simulink model "FCS_MPC_6ph_testbench_single_test"  (R2022a)
settings: Solver=ode23t  StartTime=0.0  StopTime=0.1  RelTol=1e-3  AbsTol=1e-3  EnableMultiTasking=on
values from neighbouring files (symbols this model uses):
  f_c = 100000    [Params_testbench.m]
  L_d = 0.0001473    [Params_testbench.m]
  L_q = 0.0001484    [Params_testbench.m]
  L_x = 0.00005566    (= 5.566e-05)    [Params_testbench.m]
  L_y = L_x    (= 5.566e-05)    [Params_testbench.m]
  p = 5    [Params_testbench.m]
  psi_pm = 0.0048    [Params_testbench.m]
  R_ph = 0.1278    [Params_testbench.m]
  u_dc = 36.0    (= 36)    [Params_testbench.m]
libraries: nesl_utility x39, fl_lib x32, hdlsllib x26, ee_lib x12, simulink x2, spsAlphaBetaZerotodq0Lib x1
(part 2 of 4)

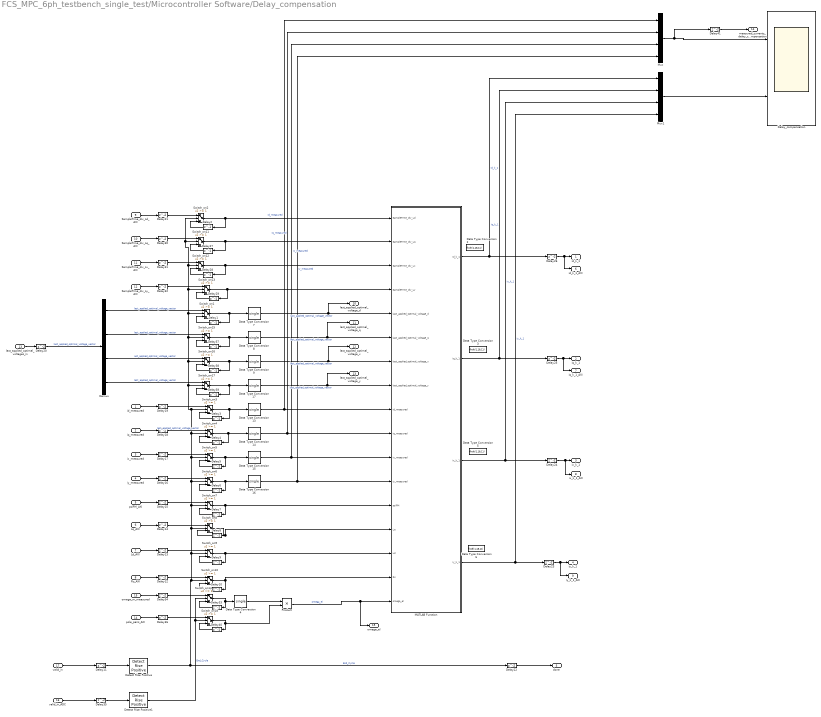
== system FCS_MPC_6ph_testbench_single_test/Microcontroller Software/Delay_compensation ==
  id_measured : Inport
  iq_measured : Inport  Port=2
  ix_measured : Inport  Port=3
  iy_measured : Inport  Port=4
  psiPM_AXI : Inport  Port=5
  Lq_AXI : Inport  Port=6
  Ld_AXI : Inport  Port=7
  Rs_AXI : Inport  Port=8
  SampleTime_div_Ld_AXI : Inport  Port=9
  SampleTime_div_Lq_AXI : Inport  Port=10
  SampleTime_div_Lx_AXI : Inport  Port=11
  SampleTime_div_Ly_AXI : Inport  Port=12
  last_applied_optimal_voltages_in : Inport  Port=13
  pole_pairs_AXI : Inport  Port=14
  omega_m_measured : Inport  Port=15
  valid_in_ADC : Inport  Port=16
  valid_in : Inport  Port=17
  Data Type Conversion{4,7..9,13..17} (9 alike) : DataTypeConversion  OutDataTypeStr=single  RndMeth=Nearest  SaturateOnIntegerOverflow=off
  Data Type Conversion{2..3,5..6} (4 alike) : DataTypeConversion  OutDataTypeStr=fixdt(1,18,11)  SaturateOnIntegerOverflow=off  RndMeth=Floor
  Delay{1..10,27..29,33,37..40} (18 alike) : Delay  DelayLength=1
  Delay{11..26,30..32,34..36,41} (23 alike) : Delay
  Delay_compensation : Scope  NumInputPorts=2
  Demux : Demux
  Detect Rise Positive : hdlsllib/Logic and Bit Operations/Detect Rise Positive  vinit=0  OutDataTypeStr=boolean
      settings: SourceProductBaseCode=SL
  Detect Rise Positive1 : hdlsllib/Logic and Bit Operations/Detect Rise Positive  vinit=0  OutDataTypeStr=boolean
      settings: SourceProductBaseCode=SL
  MATLAB Function : MATLAB Function  TreatAsAtomicUnit=on  SystemSampleTime=1/100000000
  Mux : Mux
  Mux1 : Mux
  Product : Product  Inputs=**
  Switch_on{1..18} (18 alike) : Switch  Threshold=1  RndMeth=Simplest  SaturateOnIntegerOverflow=off  InputSameDT=off  OutDataTypeStr=Inherit: Same as first input
  id_k_1 : Outport
  iq_k_1 : Outport  Port=2
  ix_k_1 : Outport  Port=3
  iy_k_1 : Outport  Port=4
  done : Outport  Port=5
  id_k_1_AXI : Outport  Port=6
  iq_k_1_AXI : Outport  Port=7
  ix_k_1_AXI : Outport  Port=8
  iy_k_1_AXI : Outport  Port=9
  last_applied_optimal_voltage_d : Outport  Port=10
  last_applied_optimal_voltage_q : Outport  Port=11
  last_applied_optimal_voltage_x : Outport  Port=12
  last_applied_optimal_voltage_y : Outport  Port=13
  measured_currents_delay_compensation : Outport  Port=14
  omega_el : Outport  Port=15
  wires:
  Switch_on14/1 -> Data Type Conversion4/1, Delay33/1
  Delay33/1 -> Switch_on14/3
  pole_pairs_AXI/1 -> Delay36/1
  Delay9/1 -> Switch_on9/3
  Switch_on9/1 -> Delay9/1, MATLAB Function/15(Ld)
  Delay32/1 -> Switch_on13/1
  Lq_AXI/1 -> Delay14/1
  Delay31/1 -> Switch_on12/1
  Switch_on12/1 -> Delay28/1, MATLAB Function/3(SampleTime_div_Lx)
  Delay30/1 -> Switch_on11/1
  Delay29/1 -> Switch_on13/3
  SampleTime_div_Lx_AXI/1 -> Delay31/1
  Delay26/1 -> id_k_1_AXI/1, id_k_1/1
  Product/1 -> omega_el/1, MATLAB Function/17(omega_el)  "omega_el"
  Delay11/1 -> Detect Rise Positive/1
  Delay2/1 -> Switch_on2/3
  SampleTime_div_Lq_AXI/1 -> Delay30/1
  Switch_on5/1 -> Delay5/1, Data Type Conversion15/1
  Delay12/1 -> Switch_on10/1
  Rs_AXI/1 -> Delay12/1
  Delay1/1 -> Switch_on1/3
  Delay27/1 -> Switch_on11/3
  Delay21/1 -> Switch_on2/1
  Delay23/1 -> iy_k_1_AXI/1, iy_k_1/1
  Delay24/1 -> ix_k_1_AXI/1, ix_k_1/1
  Delay20/1 -> Demux/1  "last_applied_optimal_voltage_vector"
  Switch_on1/1 -> Delay1/1, Data Type Conversion7/1
  Delay8/1 -> Switch_on8/3
  Delay10/1 -> Switch_on10/3
  valid_in/1 -> Delay11/1
  Switch_on6/1 -> Delay6/1, Data Type Conversion16/1
  psiPM_AXI/1 -> Delay15/1
  Delay25/1 -> iq_k_1_AXI/1, iq_k_1/1
  Switch_on13/1 -> Delay29/1, MATLAB Function/4(SampleTime_div_Ly)
  Switch_on4/1 -> Delay4/1, Data Type Conversion14/1
  Delay15/1 -> Switch_on7/1
  SampleTime_div_Ly_AXI/1 -> Delay32/1
  Switch_on10/1 -> Delay10/1, MATLAB Function/16(Rs)
  Delay7/1 -> Switch_on7/3
  Delay28/1 -> Switch_on12/3
  Switch_on8/1 -> Delay8/1, MATLAB Function/14(Lq)
  Ld_AXI/1 -> Delay13/1
  Delay6/1 -> Switch_on6/3
  Delay4/1 -> Switch_on4/3
  Switch_on11/1 -> Delay27/1, MATLAB Function/2(SampleTime_div_Lq)
  Delay3/1 -> Switch_on3/3
  Delay14/1 -> Switch_on8/1
  Switch_on2/1 -> Delay2/1, MATLAB Function/1(SampleTime_div_Ld)
  Delay22/1 -> done/1
  Switch_on3/1 -> Delay3/1, Data Type Conversion13/1
  Delay13/1 -> Switch_on9/1
  Delay5/1 -> Switch_on5/3
  SampleTime_div_Ld_AXI/1 -> Delay21/1
  last_applied_optimal_voltages_in/1 -> Delay20/1
  id_measured/1 -> Delay19/1
  iq_measured/1 -> Delay18/1
  ix_measured/1 -> Delay17/1
  iy_measured/1 -> Delay16/1
  omega_m_measured/1 -> Delay34/1
  Delay35/1 -> Detect Rise Positive1/1
  valid_in_ADC/1 -> Delay35/1
  Delay34/1 -> Switch_on14/1
  Delay36/1 -> Switch_on18/1
  Delay37/1 -> Switch_on15/3
  Delay38/1 -> Switch_on16/3
  Switch_on16/1 -> Data Type Conversion9/1, Delay38/1
  Delay39/1 -> Switch_on17/3
  Detect Rise Positive/1 -> Switch_on17/2, Switch_on16/2, Switch_on15/2, Switch_on13/2, Switch_on2/2, Switch_on11/2, Switch_on12/2, Switch_on1/2, Switch_on3/2, Switch_on4/2, Switch_on5/2, Switch_on6/2, Switch_on7/2, Switch_on8/2, Switch_on9/2, Switch_on10/2, Delay22/1  "End_Cycle"
  Switch_on17/1 -> Data Type Conversion17/1, Delay39/1
  Delay19/1 -> Switch_on3/1
  Delay18/1 -> Switch_on4/1  "last_applied_optimal_voltage_vector"
  Delay17/1 -> Switch_on5/1
  Delay16/1 -> Switch_on6/1
  Data Type Conversion4/1 -> Product/1
  MATLAB Function/1(id_k_1) -> Mux1/1, Delay26/1  "id_k_1"
  MATLAB Function/2(iq_k_1) -> Mux1/2, Delay25/1  "iq_k_1"
  MATLAB Function/3(ix_k_1) -> Mux1/3, Delay24/1  "ix_k_1"
  MATLAB Function/4(iy_k_1) -> Mux1/4, Delay23/1  "iy_k_1"
  Switch_on18/1 -> Product/2, Delay40/1
  Detect Rise Positive1/1 -> Switch_on18/2, Switch_on14/2  "End_Cycle"
  Delay40/1 -> Switch_on18/3
  Data Type Conversion13/1 -> Mux/1, MATLAB Function/9(id_measured)  "id_measured"
  Data Type Conversion14/1 -> Mux/2, MATLAB Function/10(iq_measured)  "iq_measured"
  Data Type Conversion15/1 -> Mux/3, MATLAB Function/11(ix_measured)  "ix_measured"
  Data Type Conversion16/1 -> Mux/4, MATLAB Function/12(iy_measured)  "iy_measured"
  Switch_on7/1 -> MATLAB Function/13(psiPM), Delay7/1
  Mux/1 -> Delay41/1, Delay_compensation/1
  Mux1/1 -> Delay_compensation/2
  Switch_on15/1 -> Data Type Conversion8/1, Delay37/1
  Demux/1 -> Switch_on1/1  "last_applied_optimal_voltage_vector"
  Demux/2 -> Switch_on15/1  "last_applied_optimal_voltage_vector"
  Demux/3 -> Switch_on16/1  "ast_applied_optimal_voltage_vector"
  Demux/4 -> Switch_on17/1  "last_applied_optimal_voltage_vector"
  Data Type Conversion7/1 -> last_applied_optimal_voltage_d/1, MATLAB Function/5(last_applied_optimal_voltage_d)  "last_applied_optimal_voltage_vector"
  Data Type Conversion8/1 -> last_applied_optimal_voltage_q/1, MATLAB Function/6(last_applied_optimal_voltage_q)  "last_applied_optimal_voltage_vector"
  Data Type Conversion9/1 -> last_applied_optimal_voltage_x/1, MATLAB Function/7(last_applied_optimal_voltage_x)  "last_applied_optimal_voltage_vector"
  Data Type Conversion17/1 -> last_applied_optimal_voltage_y/1, MATLAB Function/8(last_applied_optimal_voltage_y)  "last_applied_optimal_voltage_vector"
  Delay41/1 -> measured_currents_delay_compensation/1

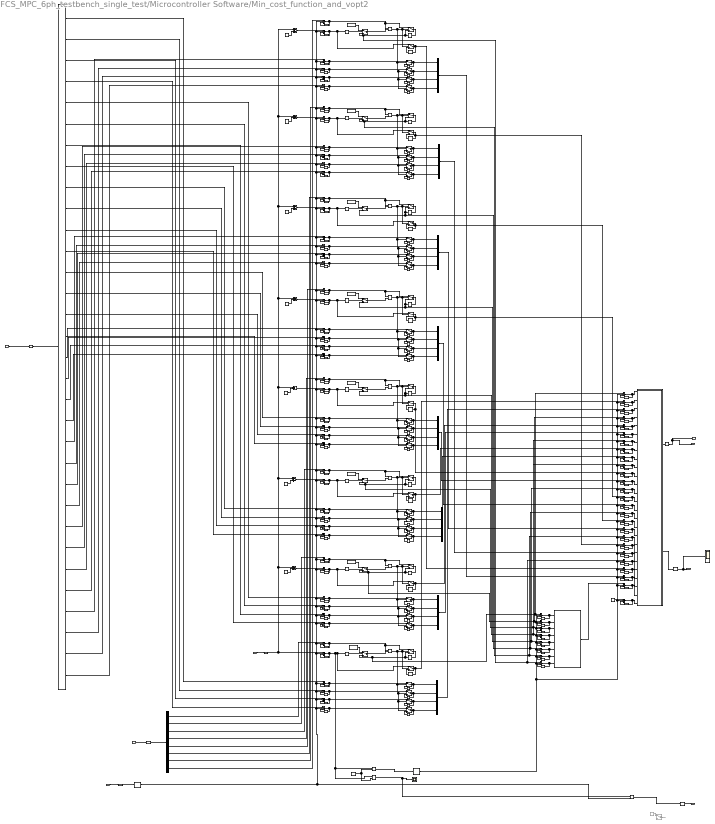
== system FCS_MPC_6ph_testbench_single_test/Microcontroller Software/Min_cost_function_and_vopt2 ==
  note: fixdt(1,24,11)
  Index_in : Inport
  valid_in : Inport  Port=2
  J_in : Inport  Port=3
  phase_voltages_per_switching_state_in : Inport  Port=4
  Add{,1..6} (7 alike) : Sum
  Compare To Constant : hdlsllib/Logic and Bit Operations/Compare To Constant  relop=<=  const=1  OutDataTypeStr=boolean
      settings: SourceProductBaseCode=SL
  Compare To Constant1 : hdlsllib/Logic and Bit Operations/Compare To Constant  relop=<=  const=9  OutDataTypeStr=boolean
      settings: SourceProductBaseCode=SL
  Compare To Constant2 : hdlsllib/Logic and Bit Operations/Compare To Constant  relop=<=  const=17  OutDataTypeStr=boolean
      settings: SourceProductBaseCode=SL
  Compare To Constant3 : hdlsllib/Logic and Bit Operations/Compare To Constant  relop=<=  const=25  OutDataTypeStr=boolean
      settings: SourceProductBaseCode=SL
  Compare To Constant4 : hdlsllib/Logic and Bit Operations/Compare To Constant  relop=<=  const=33  OutDataTypeStr=boolean
      settings: SourceProductBaseCode=SL
  Compare To Constant5 : hdlsllib/Logic and Bit Operations/Compare To Constant  relop=<=  const=41  OutDataTypeStr=boolean
      settings: SourceProductBaseCode=SL
  Compare To Constant6 : hdlsllib/Logic and Bit Operations/Compare To Constant  relop=<=  const=49  OutDataTypeStr=boolean
      settings: SourceProductBaseCode=SL
  Compare To Constant7 : hdlsllib/Logic and Bit Operations/Compare To Constant  relop=<=  const=57  OutDataTypeStr=boolean
      settings: SourceProductBaseCode=SL
  Constant{,3..9} (8 alike) : Constant  Value=1000  OutDataTypeStr=fixdt(1,20,9)  SampleTime=-1
  Constant1 : Constant  Value=8  OutDataTypeStr=int32  SampleTime=-1
  Constant11 : Constant  Value=[0;0;0;0]  OutDataTypeStr=single  SampleTime=-1
  Constant18 : Constant  Value=8  OutDataTypeStr=int32  SampleTime=-1
  Constant19 : Constant  Value=16  OutDataTypeStr=int32  SampleTime=-1
  Constant2 : Constant  Commented=on  Value=0  OutDataTypeStr=boolean  SampleTime=-1
  Constant20 : Constant  Value=24  OutDataTypeStr=int32  SampleTime=-1
  Constant21 : Constant  Value=32  OutDataTypeStr=int32  SampleTime=-1
  Constant22 : Constant  Value=40  OutDataTypeStr=int32  SampleTime=-1
  Constant23 : Constant  Value=48  OutDataTypeStr=int32  SampleTime=-1
  Constant24 : Constant  Value=56  OutDataTypeStr=int32  SampleTime=-1
  Delay{,1..5,9,15,17..73,81..90,95..96,104..113,118..119,127..136,141..142,150..159,164..165,173..182,371..378} (131 alike) : Delay  DelayLength=1
  Delay{6..8,10..12} (6 alike) : Delay
  Delay_compensation_test1 : Scope
  Demux : Demux  Outputs=8
  Demux1 : Demux  Outputs=32
  Detect Rise Positive : hdlsllib/Logic and Bit Operations/Detect Rise Positive  vinit=0  OutDataTypeStr=boolean
      settings: SourceProductBaseCode=SL
  Detect Rise Positive1 : hdlsllib/Logic and Bit Operations/Detect Rise Positive  vinit=0  OutDataTypeStr=boolean
      settings: SourceProductBaseCode=SL
  Logical Operator : Logic  AllPortsSameDT=off  OutDataTypeStr=boolean
  MATLAB Function : MATLAB Function  TreatAsAtomicUnit=on  SystemSampleTime=1/100000000
  MinMax : MinMax  Inputs=8  ZeroCross=off
  Mux{,1..7} (8 alike) : Mux
  Relational Operator{,1..8} (9 alike) : RelationalOperator  Operator=<  OutDataTypeStr=boolean  RndMeth=Simplest  InputSameDT=off
  Relational Operator9 : RelationalOperator  OutDataTypeStr=boolean  RndMeth=Simplest  InputSameDT=off
  Scope : Scope
  Switch{,1,3..6,8..9,11..14,16..21,23..28,30..35,37..42,44..49,51..56} (48 alike) : Switch  Criteria=u2 > Threshold  SaturateOnIntegerOverflow=off  InputSameDT=off  OutDataTypeStr=Inherit: Same as first input
  Switch{2,10,15,22,29,36,43,50} (8 alike) : Switch  Criteria=u2 > Threshold  OutDataTypeStr=int32  SaturateOnIntegerOverflow=off  InputSameDT=off
  Switch7 : Switch  Commented=on  Criteria=u2 > Threshold  SaturateOnIntegerOverflow=off  InputSameDT=off
  Switch_on{1..49,51..75,98..105} (82 alike) : Switch  Threshold=1  RndMeth=Simplest  SaturateOnIntegerOverflow=off  InputSameDT=off  OutDataTypeStr=Inherit: Same as first input
      Switch_on49 settings: LockScale=on
  done : Outport
  Index : Outport  Port=2
  voltages : Outport  Port=3
  Index_AXI : Outport  Port=4
  wires:
  Demux/1 -> Switch_on4/1  "End_Cycle"
  Demux1/1 -> Switch_on2/1  "End_Cycle"
  Demux1/2 -> Switch_on3/1  "End_Cycle"
  Switch5/1 -> Mux/3, Delay4/1
  Delay3/1 -> Switch4/3
  Relational Operator/1 -> Switch5/2, Switch6/2, Switch4/2, Switch3/2, Switch2/2, Switch1/2
  Compare To Constant/1 -> Switch/2
  Switch1/1 -> Delay/1
  Switch6/1 -> Delay5/1, Mux/4
  Delay4/1 -> Switch5/3
  Switch4/1 -> Mux/2, Delay3/1
  Switch/1 -> Relational Operator/2
  Delay1/1 -> Switch2/3
  Delay5/1 -> Switch6/3
  Switch3/1 -> Mux/1, Delay2/1
  Delay2/1 -> Switch3/3
  Constant/1 -> Switch/1
  Switch_on4/1 -> Relational Operator/1, Switch1/1, Delay17/1
  Switch_on1/1 -> Delay18/1, Compare To Constant/1, Switch2/1, Relational Operator9/1, Relational Operator1/1
  Switch_on2/1 -> Delay19/1, Switch3/1
  Switch_on3/1 -> Delay20/1, Switch4/1
  Switch_on5/1 -> Switch5/1, Delay21/1
  Switch_on6/1 -> Switch6/1, Delay22/1
  valid_in/1 -> Delay6/1  "End_Cycle"
  Delay17/1 -> Switch_on4/3
  Delay18/1 -> Switch_on1/3
  Delay19/1 -> Switch_on2/3
  Delay20/1 -> Switch_on3/3
  Delay21/1 -> Switch_on5/3
  Delay22/1 -> Switch_on6/3
  Constant1/1 -> Relational Operator9/2, Relational Operator1/2
  Constant2/1 -> Switch7/1
  Demux1/3 -> Switch_on5/1  "End_Cycle"
  Demux1/4 -> Switch_on6/1  "End_Cycle"
  Demux/2 -> Switch_on10/1  "End_Cycle"
  Delay34/1 -> Switch_on10/3
  Switch8/1 -> Relational Operator2/2
  Switch_on8/1 -> Delay36/1, Switch11/1
  Demux1/6 -> Switch_on9/1  "End_Cycle"
  Delay26/1 -> Switch10/3
  Add/1 -> Switch_on7/1
  Delay36/1 -> Switch_on8/3
  Delay39/1 -> Switch_on11/3
  Switch_on7/1 -> Delay35/1, Switch10/1, Compare To Constant1/1
  Compare To Constant1/1 -> Switch8/2
  Switch_on9/1 -> Delay38/1, Switch12/1
  Delay40/1 -> Switch_on12/3
  Delay35/1 -> Switch_on7/3
  Switch_on11/1 -> Switch13/1, Delay39/1
  Delay43/1 -> Switch14/3
  Switch_on12/1 -> Switch14/1, Delay40/1
  Delay37/1 -> Switch11/3
  Relational Operator2/1 -> Switch13/2, Switch14/2, Switch12/2, Switch11/2, Switch10/2, Switch9/2
  Switch9/1 -> Delay25/1
  Delay42/1 -> Switch13/3
  Demux1/5 -> Switch_on8/1  "End_Cycle"
  Demux1/7 -> Switch_on11/1  "End_Cycle"
  Switch_on10/1 -> Relational Operator2/1, Switch9/1, Delay34/1
  Demux1/8 -> Switch_on12/1  "End_Cycle"
  Delay38/1 -> Switch_on9/3
  Constant3/1 -> Switch8/1
  Delay41/1 -> Switch12/3
  Delay61/1 -> Switch16/3
  Switch_on16/1 -> Switch19/1, Delay64/1
  Delay67/1 -> Switch19/3
  Switch_on15/1 -> Switch18/1, Delay63/1
  Delay59/1 -> Switch_on17/3
  Switch_on19/1 -> Delay62/1, Switch17/1
  Delay64/1 -> Switch_on16/3
  Switch_on17/1 -> Delay59/1, Switch15/1, Compare To Constant2/1
  Compare To Constant2/1 -> Switch20/2
  Demux1/10 -> Switch_on19/1  "End_Cycle"
  Delay50/1 -> Switch15/3
  Switch20/1 -> Relational Operator3/2
  Demux/3 -> Switch_on14/1  "End_Cycle"
  Delay65/1 -> Switch17/3
  Switch_on14/1 -> Relational Operator3/1, Switch21/1, Delay58/1
  Switch_on18/1 -> Delay60/1, Switch16/1
  Constant4/1 -> Switch20/1
  Demux1/11 -> Switch_on15/1  "End_Cycle"
  Delay63/1 -> Switch_on15/3
  Delay66/1 -> Switch18/3
  Switch21/1 -> Delay49/1
  Demux1/9 -> Switch_on18/1  "End_Cycle"
  Demux1/12 -> Switch_on16/1  "End_Cycle"
  Add1/1 -> Switch_on17/1
  Delay60/1 -> Switch_on18/3
  Relational Operator3/1 -> Switch18/2, Switch19/2, Switch17/2, Switch16/2, Switch15/2, Switch21/2
  Delay58/1 -> Switch_on14/3
  Delay62/1 -> Switch_on19/3
  Delay84/1 -> Switch23/3
  Switch_on22/1 -> Switch26/1, Delay87/1
  Delay90/1 -> Switch26/3
  Switch_on21/1 -> Switch25/1, Delay86/1
  Delay82/1 -> Switch_on23/3
  Switch_on25/1 -> Delay85/1, Switch24/1
  Delay87/1 -> Switch_on22/3
  Switch_on23/1 -> Delay82/1, Switch22/1, Compare To Constant3/1
  Compare To Constant3/1 -> Switch27/2
  Demux1/14 -> Switch_on25/1  "End_Cycle"
  Delay73/1 -> Switch22/3
  Switch27/1 -> Relational Operator4/2
  Demux/4 -> Switch_on20/1  "End_Cycle"
  Delay88/1 -> Switch24/3
  Switch_on20/1 -> Relational Operator4/1, Switch28/1, Delay81/1
  Switch_on24/1 -> Delay83/1, Switch23/1
  Constant5/1 -> Switch27/1
  Demux1/15 -> Switch_on21/1  "End_Cycle"
  Delay86/1 -> Switch_on21/3
  Delay89/1 -> Switch25/3
  Switch28/1 -> Delay72/1
  Demux1/13 -> Switch_on24/1  "End_Cycle"
  Demux1/16 -> Switch_on22/1  "End_Cycle"
  Add2/1 -> Switch_on23/1
  Delay83/1 -> Switch_on24/3
  Relational Operator4/1 -> Switch25/2, Switch26/2, Switch24/2, Switch23/2, Switch22/2, Switch28/2
  Delay81/1 -> Switch_on20/3
  Delay85/1 -> Switch_on25/3
  Delay107/1 -> Switch30/3
  Switch_on28/1 -> Switch33/1, Delay110/1
  Delay113/1 -> Switch33/3
  Switch_on27/1 -> Switch32/1, Delay109/1
  Delay105/1 -> Switch_on29/3
  Switch_on31/1 -> Delay108/1, Switch31/1
  Delay110/1 -> Switch_on28/3
  Switch_on29/1 -> Delay105/1, Switch29/1, Compare To Constant4/1
  Compare To Constant4/1 -> Switch34/2
  Demux1/18 -> Switch_on31/1  "End_Cycle"
  Delay96/1 -> Switch29/3
  Switch34/1 -> Relational Operator5/2
  Demux/5 -> Switch_on26/1  "End_Cycle"
  Delay111/1 -> Switch31/3
  Switch_on26/1 -> Relational Operator5/1, Switch35/1, Delay104/1
  Switch_on30/1 -> Delay106/1, Switch30/1
  Constant6/1 -> Switch34/1
  Demux1/19 -> Switch_on27/1  "End_Cycle"
  Delay109/1 -> Switch_on27/3
  Delay112/1 -> Switch32/3
  Switch35/1 -> Delay95/1
  Demux1/17 -> Switch_on30/1  "End_Cycle"
  Demux1/20 -> Switch_on28/1  "End_Cycle"
  Add3/1 -> Switch_on29/1
  Delay106/1 -> Switch_on30/3
  Relational Operator5/1 -> Switch32/2, Switch33/2, Switch31/2, Switch30/2, Switch29/2, Switch35/2
  Delay104/1 -> Switch_on26/3
  Delay108/1 -> Switch_on31/3
  Delay130/1 -> Switch37/3
  Switch_on34/1 -> Switch40/1, Delay133/1
  Delay136/1 -> Switch40/3
  Switch_on33/1 -> Switch39/1, Delay132/1
  Delay128/1 -> Switch_on35/3
  Switch_on37/1 -> Delay131/1, Switch38/1
  Delay133/1 -> Switch_on34/3
  Switch_on35/1 -> Delay128/1, Switch36/1, Compare To Constant5/1
  Compare To Constant5/1 -> Switch41/2
  Demux1/22 -> Switch_on37/1  "End_Cycle"
  Delay119/1 -> Switch36/3
  Switch41/1 -> Relational Operator6/2
  Demux/6 -> Switch_on32/1  "End_Cycle"
  Delay134/1 -> Switch38/3
  Switch_on32/1 -> Relational Operator6/1, Switch42/1, Delay127/1
  Switch_on36/1 -> Delay129/1, Switch37/1
  Constant7/1 -> Switch41/1
  Demux1/23 -> Switch_on33/1  "End_Cycle"
  Delay132/1 -> Switch_on33/3
  Delay135/1 -> Switch39/3
  Switch42/1 -> Delay118/1
  Demux1/21 -> Switch_on36/1  "End_Cycle"
  Demux1/24 -> Switch_on34/1  "End_Cycle"
  Add4/1 -> Switch_on35/1
  Delay129/1 -> Switch_on36/3
  Relational Operator6/1 -> Switch39/2, Switch40/2, Switch38/2, Switch37/2, Switch36/2, Switch42/2
  Delay127/1 -> Switch_on32/3
  Delay131/1 -> Switch_on37/3
  Delay153/1 -> Switch44/3
  Switch_on40/1 -> Switch47/1, Delay156/1
  Delay159/1 -> Switch47/3
  Switch_on39/1 -> Switch46/1, Delay155/1
  Delay151/1 -> Switch_on41/3
  Switch_on43/1 -> Delay154/1, Switch45/1
  Delay156/1 -> Switch_on40/3
  Switch_on41/1 -> Delay151/1, Switch43/1, Compare To Constant6/1
  Compare To Constant6/1 -> Switch48/2
  Demux1/26 -> Switch_on43/1  "End_Cycle"
  Delay142/1 -> Switch43/3
  Switch48/1 -> Relational Operator7/2
  Delay157/1 -> Switch45/3
  Switch_on38/1 -> Relational Operator7/1, Switch49/1, Delay150/1
  Switch_on42/1 -> Delay152/1, Switch44/1
  Constant8/1 -> Switch48/1
  Demux1/27 -> Switch_on39/1  "End_Cycle"
  Delay155/1 -> Switch_on39/3
  Delay158/1 -> Switch46/3
  Switch49/1 -> Delay141/1
  Demux1/25 -> Switch_on42/1  "End_Cycle"
  Demux1/28 -> Switch_on40/1  "End_Cycle"
  Add5/1 -> Switch_on41/1
  Delay152/1 -> Switch_on42/3
  Relational Operator7/1 -> Switch46/2, Switch47/2, Switch45/2, Switch44/2, Switch43/2, Switch49/2
  Delay150/1 -> Switch_on38/3
  Delay154/1 -> Switch_on43/3
  Delay176/1 -> Switch51/3
  Switch_on46/1 -> Switch54/1, Delay179/1
  Delay182/1 -> Switch54/3
  Switch_on45/1 -> Switch53/1, Delay178/1
  Delay174/1 -> Switch_on47/3
  Switch_on49/1 -> Delay177/1, Switch52/1
  Delay179/1 -> Switch_on46/3
  Switch_on47/1 -> Delay174/1, Switch50/1, Compare To Constant7/1
  Compare To Constant7/1 -> Switch55/2
  Demux1/30 -> Switch_on49/1  "End_Cycle"
  Delay165/1 -> Switch50/3
  Switch55/1 -> Relational Operator8/2
  Demux/8 -> Switch_on44/1  "End_Cycle"
  Delay180/1 -> Switch52/3
  Switch_on44/1 -> Relational Operator8/1, Switch56/1, Delay173/1
  Switch_on48/1 -> Delay175/1, Switch51/1
  Constant9/1 -> Switch55/1
  Demux1/31 -> Switch_on45/1  "End_Cycle"
  Delay178/1 -> Switch_on45/3
  Delay181/1 -> Switch53/3
  Switch56/1 -> Delay164/1
  Demux1/29 -> Switch_on48/1  "End_Cycle"
  Demux1/32 -> Switch_on46/1  "End_Cycle"
  Add6/1 -> Switch_on47/1
  Delay175/1 -> Switch_on48/3
  Relational Operator8/1 -> Switch53/2, Switch54/2, Switch52/2, Switch51/2, Switch50/2, Switch56/2
  Delay173/1 -> Switch_on44/3
  Delay177/1 -> Switch_on49/3
  Detect Rise Positive/1 -> Logical Operator/2, Switch_on44/2, Switch_on47/2, Switch_on48/2, Switch_on49/2, Switch_on45/2, Switch_on46/2, Switch_on38/2, Switch_on41/2, Switch_on42/2, Switch_on43/2, Switch_on39/2, Switch_on40/2, Switch_on32/2, Switch_on35/2, Switch_on36/2, Switch_on37/2, Switch_on33/2, Switch_on34/2, Switch_on26/2, Switch_on29/2, Switch_on30/2, Switch_on31/2, Switch_on27/2, Switch_on28/2, Switch_on20/2, Switch_on23/2, Switch_on24/2, Switch_on25/2, Switch_on21/2, Switch_on22/2, Switch_on14/2, Switch_on17/2, Switch_on18/2, Switch_on19/2, Switch_on15/2, Switch_on16/2, Switch_on10/2, Switch_on7/2, Switch_on8/2, Switch_on9/2, Switch_on11/2, Switch_on12/2, Switch_on4/2, Switch_on1/2, Switch_on2/2, Switch_on3/2, Switch_on5/2, Switch_on6/2  "End_Cycle"
  Constant18/1 -> Add/2
  Constant19/1 -> Add1/2
  Constant20/1 -> Add2/2
  Constant21/1 -> Add3/2
  Constant22/1 -> Add4/2
  Constant23/1 -> Add5/2
  Constant24/1 -> Add6/2
  Delay371/1 -> Switch_on98/3
  Switch_on98/1 -> Delay371/1, MinMax/1
  Switch_on99/1 -> Delay372/1, MinMax/2
  Delay372/1 -> Switch_on99/3
  Switch_on100/1 -> Delay373/1, MinMax/3
  Delay373/1 -> Switch_on100/3
  Switch_on101/1 -> Delay374/1, MinMax/4
  Delay374/1 -> Switch_on101/3
  Delay376/1 -> Switch_on105/3
  Switch_on102/1 -> Delay377/1, MinMax/7
  Delay377/1 -> Switch_on102/3
  Switch_on104/1 -> Delay375/1, MinMax/5
  Delay375/1 -> Switch_on104/3
  Switch_on105/1 -> Delay376/1, MinMax/6
  Switch_on103/1 -> Delay378/1, MinMax/8
  Delay378/1 -> Switch_on103/3
  Relational Operator1/1 -> Logical Operator/1, Scope/1  "End_Cycle"
  Switch13/1 -> Mux1/3, Delay42/1
  Switch12/1 -> Mux1/2, Delay41/1
  Switch14/1 -> Mux1/4, Delay43/1
  Switch11/1 -> Mux1/1, Delay37/1
  Switch18/1 -> Mux2/3, Delay66/1
  Switch17/1 -> Mux2/2, Delay65/1
  Switch19/1 -> Mux2/4, Delay67/1
  Switch16/1 -> Mux2/1, Delay61/1
  Switch25/1 -> Delay89/1, Mux3/3
  Switch24/1 -> Mux3/2, Delay88/1
  Switch26/1 -> Mux3/4, Delay90/1
  Switch23/1 -> Mux3/1, Delay84/1
  Switch32/1 -> Mux4/3, Delay112/1
  Switch31/1 -> Mux4/2, Delay111/1
  Switch33/1 -> Mux4/4, Delay113/1
  Switch30/1 -> Delay107/1, Mux4/1
  Switch39/1 -> Mux5/3, Delay135/1
  Switch38/1 -> Delay134/1, Mux5/2
  Switch40/1 -> Mux5/4, Delay136/1
  Switch37/1 -> Mux5/1, Delay130/1
  Switch46/1 -> Mux6/3, Delay158/1
  Switch45/1 -> Mux6/2, Delay157/1
  Switch47/1 -> Mux6/4, Delay159/1
  Switch44/1 -> Mux6/1, Delay153/1
  Switch53/1 -> Mux7/3, Delay181/1
  Switch52/1 -> Mux7/2, Delay180/1
  Switch54/1 -> Mux7/4, Delay182/1
  Switch51/1 -> Mux7/1, Delay176/1
  Demux/7 -> Switch_on38/1  "End_Cycle"
  J_in/1 -> Delay7/1  "End_Cycle"
  phase_voltages_per_switching_state_in/1 -> Delay8/1  "End_Cycle"
  Logical Operator/1 -> Delay12/1
  Delay6/1 -> Detect Rise Positive/1
  Delay7/1 -> Demux/1
  Delay8/1 -> Demux1/1
  Index_in/1 -> Delay9/1
  Switch7/1 -> ?
  MATLAB Function/2(voltages) -> Delay11/1
  MATLAB Function/1(Index) -> Delay10/1
  Constant11/1 -> Switch_on13/1
  Switch_on13/1 -> MATLAB Function/26(voltages_default), Delay15/1
  Delay15/1 -> Switch_on13/3
  Switch_on51/1 -> MATLAB Function/25(min), Delay23/1
  Delay23/1 -> Switch_on51/3
  Switch_on52/1 -> MATLAB Function/24(voltages_8), Delay24/1
  Delay24/1 -> Switch_on52/3
  Switch50/1 -> Switch_on53/1, Delay165/1
  Switch_on53/1 -> MATLAB Function/23(Index_8), Delay27/1
  Delay27/1 -> Switch_on53/3
  Switch_on54/1 -> MATLAB Function/22(J_8), Delay28/1
  Delay28/1 -> Switch_on54/3
  Switch_on55/1 -> MATLAB Function/21(voltages_7), Delay29/1
  Delay29/1 -> Switch_on55/3
  Switch43/1 -> Switch_on56/1, Delay142/1
  Switch_on56/1 -> MATLAB Function/20(Index_7), Delay30/1
  Delay30/1 -> Switch_on56/3
  Switch_on57/1 -> MATLAB Function/19(J_7), Delay31/1
  Delay31/1 -> Switch_on57/3
  Switch_on58/1 -> MATLAB Function/18(voltages_6), Delay32/1
  Delay32/1 -> Switch_on58/3
  Switch36/1 -> Switch_on59/1, Delay119/1
  Switch_on59/1 -> MATLAB Function/17(Index_6), Delay33/1
  Delay33/1 -> Switch_on59/3
  Switch_on60/1 -> MATLAB Function/16(J_6), Delay44/1
  Delay44/1 -> Switch_on60/3
  Switch_on61/1 -> MATLAB Function/15(voltages_5), Delay45/1
  Delay45/1 -> Switch_on61/3
  Switch29/1 -> Switch_on62/1, Delay96/1
  Switch_on62/1 -> MATLAB Function/14(Index_5), Delay46/1
  Delay46/1 -> Switch_on62/3
  Switch_on63/1 -> MATLAB Function/13(J_5), Delay47/1
  Delay47/1 -> Switch_on63/3
  Switch_on64/1 -> MATLAB Function/12(voltages_4), Delay48/1
  Delay48/1 -> Switch_on64/3
  Switch22/1 -> Switch_on65/1, Delay73/1
  Switch_on65/1 -> MATLAB Function/11(Index_4), Delay51/1
  Delay51/1 -> Switch_on65/3
  Switch_on66/1 -> MATLAB Function/10(J_4), Delay52/1
  Delay52/1 -> Switch_on66/3
  Switch_on67/1 -> MATLAB Function/9(voltages_3), Delay53/1
  Delay53/1 -> Switch_on67/3
  Switch15/1 -> Switch_on68/1, Delay50/1
  Switch_on68/1 -> MATLAB Function/8(Index_3), Delay54/1
  Delay54/1 -> Switch_on68/3
  Switch_on69/1 -> MATLAB Function/7(J_3), Delay55/1
  Delay55/1 -> Switch_on69/3
  Switch_on70/1 -> MATLAB Function/6(voltages_2), Delay56/1
  Delay56/1 -> Switch_on70/3
  Switch10/1 -> Switch_on71/1, Delay26/1
  Switch_on71/1 -> MATLAB Function/5(Index_2), Delay57/1
  Delay57/1 -> Switch_on71/3
  Switch_on72/1 -> MATLAB Function/4(J_2), Delay68/1
  Delay68/1 -> Switch_on72/3
  Switch_on73/1 -> MATLAB Function/3(voltages_1), Delay69/1
  Delay69/1 -> Switch_on73/3
  Switch2/1 -> Switch_on74/1, Delay1/1
  Switch_on74/1 -> MATLAB Function/2(Index_1), Delay70/1
  Delay70/1 -> Switch_on74/3
  Switch_on75/1 -> MATLAB Function/1(J_1), Delay71/1
  Delay71/1 -> Switch_on75/3
  Delay/1 -> Switch_on75/1, Switch_on98/1, Switch/3, Switch1/3  "last_applied_optimal_voltage_vector"
  Mux/1 -> Switch_on73/1  "last_applied_optimal_voltage_vector"
  Delay25/1 -> Switch_on72/1, Switch_on99/1, Switch8/3, Switch9/3  "last_applied_optimal_voltage_vector"
  Mux1/1 -> Switch_on70/1  "last_applied_optimal_voltage_vector"
  Delay49/1 -> Switch_on69/1, Switch_on100/1, Switch20/3, Switch21/3  "last_applied_optimal_voltage_vector"
  Mux2/1 -> Switch_on67/1  "last_applied_optimal_voltage_vector"
  Delay72/1 -> Switch_on66/1, Switch_on101/1, Switch27/3, Switch28/3  "last_applied_optimal_voltage_vector"
  Mux3/1 -> Switch_on64/1  "last_applied_optimal_voltage_vector"
  Delay95/1 -> Switch34/3, Switch_on63/1, Switch_on104/1, Switch35/3  "last_applied_optimal_voltage_vector"
  Mux4/1 -> Switch_on61/1  "last_applied_optimal_voltage_vector"
  Delay118/1 -> Switch41/3, Switch_on60/1, Switch_on105/1, Switch42/3  "last_applied_optimal_voltage_vector"
  Mux5/1 -> Switch_on58/1  "last_applied_optimal_voltage_vector"
  Delay141/1 -> Switch_on57/1, Switch_on102/1, Switch48/3, Switch49/3  "last_applied_optimal_voltage_vector"
  Mux6/1 -> Switch_on55/1  "last_applied_optimal_voltage_vector"
  Delay164/1 -> Switch_on54/1, Switch_on103/1, Switch55/3, Switch56/3  "last_applied_optimal_voltage_vector"
  Mux7/1 -> Switch_on52/1  "last_applied_optimal_voltage_vector"
  MinMax/1 -> Switch_on51/1  "last_applied_optimal_voltage_vector"
  Delay10/1 -> Index_AXI/1, Index/1
  Delay11/1 -> Delay_compensation_test1/1, voltages/1
  Delay12/1 -> done/1
  Detect Rise Positive1/1 -> Switch_on52/2, Switch_on53/2, Switch_on75/2, Switch_on74/2, Switch_on73/2, Switch_on72/2, Switch_on71/2, Switch_on70/2, Switch_on69/2, Switch_on68/2, Switch_on67/2, Switch_on66/2, Switch_on65/2, Switch_on64/2, Switch_on63/2, Switch_on62/2, Switch_on61/2, Switch_on60/2, Switch_on59/2, Switch_on58/2, Switch_on57/2, Switch_on56/2, Switch_on55/2, Switch_on54/2, Switch_on51/2, Switch_on13/2, Switch_on98/2, Switch_on99/2, Switch_on100/2, Switch_on101/2, Switch_on104/2, Switch_on105/2, Switch_on102/2, Switch_on103/2  "End_Cycle"
  Relational Operator9/1 -> Detect Rise Positive1/1  "End_Cycle"
  Delay9/1 -> Switch_on1/1, Add/1, Add3/1, Add6/1, Add5/1, Add4/1, Add2/1, Add1/1

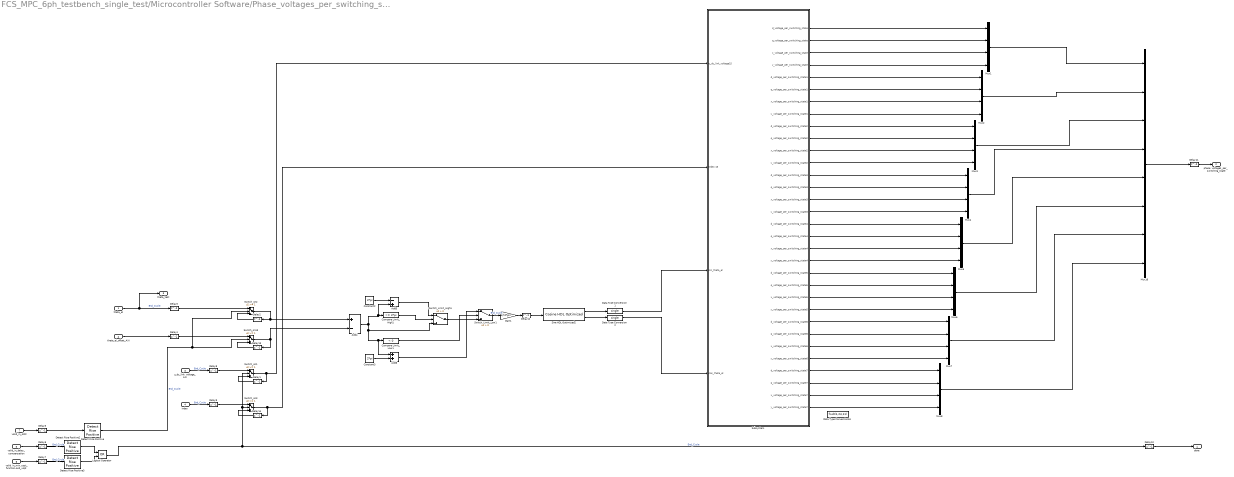
== system FCS_MPC_6ph_testbench_single_test/Microcontroller Software/Phase_voltages_per_switching_state2 ==
  theta_el : Inport
  theta_el_offset_AXI : Inport  Port=2
  u_dc_link_voltage_AXI : Inport  Port=3
  Index : Inport  Port=4
  valid_in_delay_compensation : Inport  Port=5
  valid_in_min_cost_function-and_vopt : Inport  Port=6
  valid_in_ADC : Inport  Port=7
  Add4 : Sum  Inputs=+-  OutDataTypeStr=Inherit: Same as first input
  Add5 : Sum  Inputs=-+  OutDataTypeStr=Inherit: Same as first input
  Add6 : Sum  OutDataTypeStr=Inherit: Same as first input
  Compare Limit_High1 : simulink/Logic and Bit Operations/Compare To Constant  relop=>=  const=2*pi  OutDataTypeStr=boolean
  Compare Limit_Low1 : simulink/Logic and Bit Operations/Compare To Constant  relop=<  const=0  OutDataTypeStr=boolean
  Constant2 : Constant  Value=2*pi  OutDataTypeStr=fixdt(1,24,20)  SampleTime=1/100000000
  Constant3 : Constant  Value=2*pi  OutDataTypeStr=fixdt(1,24,20)  SampleTime=1/100000000
  Data Type Conversion1 : DataTypeConversion  OutDataTypeStr=single  SaturateOnIntegerOverflow=off  RndMeth=Floor
  Data Type Conversion2 : DataTypeConversion  OutDataTypeStr=single  SaturateOnIntegerOverflow=off  RndMeth=Floor
  Data Type Conversion34 : DataTypeConversion  OutDataTypeStr=fixdt(1,24,11)  SaturateOnIntegerOverflow=off  RndMeth=Floor
  Delay{1..14} (14 alike) : Delay  DelayLength=1
  Detect Rise Positive : hdlsllib/Logic and Bit Operations/Detect Rise Positive  vinit=0  OutDataTypeStr=boolean
      settings: SourceProductBaseCode=SL
  Detect Rise Positive2 : hdlsllib/Logic and Bit Operations/Detect Rise Positive  vinit=0  OutDataTypeStr=boolean
      settings: SourceProductBaseCode=SL
  Detect Rise Positive3 : hdlsllib/Logic and Bit Operations/Detect Rise Positive  vinit=0  OutDataTypeStr=boolean
      settings: SourceProductBaseCode=SL
  Gain1 : Gain  Gain=1/(2*pi)  OutDataTypeStr=Inherit: Same as input  ParamDataTypeStr=Inherit: Same as input
  Logical Operator : Logic  Operator=OR  AllPortsSameDT=off  OutDataTypeStr=boolean
  Mux{1..8} (8 alike) : Mux
  Mux16 : Mux  Inputs=8
  Sine HDL Optimized2 : hdlsllib/Lookup Tables/Cosine HDL Optimized  OutputFormula=sin(2*pi*u) and cos(2*pi*u)  NumDataPoints=1024  TableDataTypeStr=fixdt(1,23,20)  SimulateLUTROMDelay=off
      settings: SourceProductBaseCode=SL
  Subsystem : Subsystem
  Switch_Limit_High1 : Switch  Criteria=u2 > Threshold  SaturateOnIntegerOverflow=off  InputSameDT=off  OutDataTypeStr=Inherit: Same as first input
  Switch_Limit_Low1 : Switch  Criteria=u2 > Threshold  SaturateOnIntegerOverflow=off  InputSameDT=off  OutDataTypeStr=Inherit: Same as first input
  Switch_on1 : Switch  Threshold=1  OutDataTypeStr=single  RndMeth=Simplest  SaturateOnIntegerOverflow=off  InputSameDT=off
  Switch_on13 : Switch  Threshold=1  RndMeth=Simplest  SaturateOnIntegerOverflow=off  InputSameDT=off  OutDataTypeStr=Inherit: Same as first input
  Switch_on2 : Switch  Threshold=1  RndMeth=Simplest  SaturateOnIntegerOverflow=off  InputSameDT=off  OutDataTypeStr=Inherit: Same as first input
  Switch_on3 : Switch  Threshold=1  OutDataTypeStr=int32  RndMeth=Simplest  SaturateOnIntegerOverflow=off  InputSameDT=off
  done : Outport
  phase_voltages_per_switching_state : Outport  Port=2
  theta_test : Outport  Port=3
  wires:
  Delay14/1 -> Switch_on3/3
  Delay13/1 -> Switch_on13/3
  Switch_on13/1 -> Delay13/1, Add4/2
  u_dc_link_voltage_AXI/1 -> Delay8/1  "End_Cycle"
  Switch_on1/1 -> Subsystem/1(u_dc_link_voltage15), Delay1/1
  Logical Operator/1 -> Delay10/1, Switch_on3/2, Switch_on1/2  "End_Cycle"
  Delay1/1 -> Switch_on1/3
  Index/1 -> Delay9/1  "End_Cycle"
  Switch_on3/1 -> Delay14/1, Subsystem/2(Index 15)
  Mux1/1 -> Mux16/1
  Mux2/1 -> Mux16/2
  Mux3/1 -> Mux16/3
  Mux4/1 -> Mux16/4
  Mux5/1 -> Mux16/5
  Mux6/1 -> Mux16/6
  Mux7/1 -> Mux16/7
  Mux8/1 -> Mux16/8
  Mux16/1 -> Delay11/1
  valid_in_ADC/1 -> Delay5/1
  valid_in_delay_compensation/1 -> Delay6/1
  valid_in_min_cost_function-and_vopt/1 -> Delay7/1
  theta_el/1 -> theta_test/1, Delay3/1  "End_Cycle"
  Add4/1 -> Switch_Limit_High1/3, Add6/1, Compare Limit_Low1/1, Add5/2, Compare Limit_High1/1
  Compare Limit_Low1/1 -> Switch_Limit_Low1/2
  Add5/1 -> Switch_Limit_High1/1
  theta_el_offset_AXI/1 -> Delay4/1
  Constant3/1 -> Add6/2
  Constant2/1 -> Add5/1
  Compare Limit_High1/1 -> Switch_Limit_High1/2
  Add6/1 -> Switch_Limit_Low1/1
  Switch_Limit_High1/1 -> Switch_Limit_Low1/3
  Delay2/1 -> Switch_on2/3
  Switch_on2/1 -> Add4/1, Delay2/1
  Detect Rise Positive/1 -> Switch_on2/2, Switch_on13/2  "End_Cycle"
  Delay3/1 -> Switch_on2/1
  Delay4/1 -> Switch_on13/1
  Delay5/1 -> Detect Rise Positive/1
  Delay6/1 -> Detect Rise Positive2/1
  Delay7/1 -> Detect Rise Positive3/1
  Delay8/1 -> Switch_on1/1
  Delay9/1 -> Switch_on3/1
  Delay10/1 -> done/1
  Delay11/1 -> phase_voltages_per_switching_state/1
  Sine HDL Optimized2/2 -> Data Type Conversion2/1
  Sine HDL Optimized2/1 -> Data Type Conversion1/1
  Data Type Conversion2/1 -> Subsystem/4(cos_theta_el)
  Data Type Conversion1/1 -> Subsystem/3(sin_theta_el)
  Gain1/1 -> Delay12/1
  Delay12/1 -> Sine HDL Optimized2/1
  Switch_Limit_Low1/1 -> Gain1/1  "End_Cycle"
  Subsystem/1(d_voltage_per_switching_state) -> Mux1/1
  Subsystem/2(q_voltage_per_switching_state) -> Mux1/2
  Subsystem/3(x_voltage_per_switching_state) -> Mux1/3
  Subsystem/4(y_voltage_per_switching_state) -> Mux1/4
  Subsystem/5(d_voltage_per_switching_state1) -> Mux2/1
  Subsystem/6(q_voltage_per_switching_state1) -> Mux2/2
  Subsystem/7(x_voltage_per_switching_state1) -> Mux2/3
  Subsystem/8(y_voltage_per_switching_state1) -> Mux2/4
  Subsystem/9(d_voltage_per_switching_state2) -> Mux3/1
  Subsystem/10(q_voltage_per_switching_state2) -> Mux3/2
  Subsystem/11(x_voltage_per_switching_state2) -> Mux3/3
  Subsystem/12(y_voltage_per_switching_state2) -> Mux3/4
  Subsystem/13(d_voltage_per_switching_state3) -> Mux4/1
  Subsystem/14(q_voltage_per_switching_state3) -> Mux4/2
  Subsystem/15(x_voltage_per_switching_state3) -> Mux4/3
  Subsystem/16(y_voltage_per_switching_state3) -> Mux4/4
  Subsystem/17(d_voltage_per_switching_state4) -> Mux5/1
  Subsystem/18(q_voltage_per_switching_state4) -> Mux5/2
  Subsystem/19(x_voltage_per_switching_state4) -> Mux5/3
  Subsystem/20(y_voltage_per_switching_state4) -> Mux5/4
  Subsystem/21(d_voltage_per_switching_state5) -> Mux6/1
  Subsystem/22(q_voltage_per_switching_state5) -> Mux6/2
  Subsystem/23(x_voltage_per_switching_state5) -> Mux6/3
  Subsystem/24(y_voltage_per_switching_state5) -> Mux6/4
  Subsystem/25(d_voltage_per_switching_state6) -> Mux7/1
  Subsystem/26(q_voltage_per_switching_state6) -> Mux7/2
  Subsystem/27(x_voltage_per_switching_state6) -> Mux7/3
  Subsystem/28(y_voltage_per_switching_state6) -> Mux7/4
  Subsystem/29(d_voltage_per_switching_state7) -> Mux8/1
  Subsystem/30(q_voltage_per_switching_state7) -> Mux8/2
  Subsystem/31(x_voltage_per_switching_state7) -> Mux8/3
  Subsystem/32(y_voltage_per_switching_state7) -> Mux8/4
  Detect Rise Positive2/1 -> Logical Operator/1  "End_Cycle"
  Detect Rise Positive3/1 -> Logical Operator/2  "End_Cycle"
